simulink model "MIL_ASW"  (R2019b)
settings: Solver=FixedStepDiscrete  StartTime=0.0  StopTime=2  FixedStep=0.001  RelTol=1e-3  EnableMultiTasking=on
model workspace (MAT data in the model file):
  AccPedlCanVal : Simulink.Signal (value not decoded)
  AccPedlVal : Simulink.Signal (value not decoded)
  BrkPedlCanVal : Simulink.Signal (value not decoded)
  BrkPedlVal : Simulink.Signal (value not decoded)
  Cal1 : Simulink.Parameter (value not decoded)
  Cal10 : Simulink.Parameter (value not decoded)
  Cal11 : Simulink.Parameter (value not decoded)
  Cal12 : Simulink.Parameter (value not decoded)
  Cal2 : Simulink.Parameter (value not decoded)
  Cal3 : Simulink.Parameter (value not decoded)
  Cal4 : Simulink.Parameter (value not decoded)
  Cal5 : Simulink.Parameter (value not decoded)
  Cal6 : Simulink.Parameter (value not decoded)
  Cal7 : Simulink.Parameter (value not decoded)
  Cal8 : Simulink.Parameter (value not decoded)
  Cal9 : Simulink.Parameter (value not decoded)
  Clu1Act : Simulink.Signal (value not decoded)
  Clu1PTar : Simulink.Signal (value not decoded)
  Clu1Req : Simulink.Signal (value not decoded)
  Clu1TqTar : Simulink.Signal (value not decoded)
  Clu2Act : Simulink.Signal (value not decoded)
  Clu2PTar : Simulink.Signal (value not decoded)
  Clu2Req : Simulink.Signal (value not decoded)
  Clu2TqTar : Simulink.Signal (value not decoded)
  CluKissPtPLnch : Simulink.Parameter (value not decoded)
  CluOilTRawVal : Simulink.Signal (value not decoded)
  CluOilTVal : Simulink.Signal (value not decoded)
  CluOpenTqRatMax : Simulink.Parameter (value not decoded)
  CluPMap : Simulink.Parameter (value not decoded)
  CluPMax : Simulink.Parameter (value not decoded)
  CluPMaxGear1 : Simulink.Parameter (value not decoded)
  CluPMaxGear2 : Simulink.Parameter (value not decoded)
  CluPMaxGear3 : Simulink.Parameter (value not decoded)
  CluPMaxGear4 : Simulink.Parameter (value not decoded)
  CluPMaxGear5 : Simulink.Parameter (value not decoded)
  CluPMaxGear6 : Simulink.Parameter (value not decoded)
  CluPMaxGearR : Simulink.Parameter (value not decoded)
  CluPMin : Simulink.Parameter (value not decoded)
  CluPosnMax : Simulink.Parameter (value not decoded)
  CluSoln1IRawVal : Simulink.Signal (value not decoded)
  CluSoln1IReq : Simulink.Signal (value not decoded)
  CluSoln1IReqFlg : Simulink.Signal (value not decoded)
  CluSoln1IVal : Simulink.Signal (value not decoded)
  CluSoln1LineI : Simulink.Parameter (value not decoded)
  CluSoln1LineP : Simulink.Parameter (value not decoded)
  CluSoln1Pwm : Simulink.Signal (value not decoded)
  CluSoln2IRawVal : Simulink.Signal (value not decoded)
  CluSoln2IReq : Simulink.Signal (value not decoded)
  CluSoln2IReqFlg : Simulink.Signal (value not decoded)
  CluSoln2IVal : Simulink.Signal (value not decoded)
  CluSoln2LineI : Simulink.Parameter (value not decoded)
  CluSoln2LineP : Simulink.Parameter (value not decoded)
  CluSoln2Pwm : Simulink.Signal (value not decoded)
  CluTqMap : Simulink.Parameter (value not decoded)
  CrnkSpdRawVal : Simulink.Signal (value not decoded)
  CrnkSpdVal : Simulink.Signal (value not decoded)
  Drive_Intensity_Fuzzy : object (value not decoded)
  DrvIntenFzzy : Simulink.LookupTable (value not decoded)
  EngNIdle : Simulink.Parameter (value not decoded)
  EngNIdleMin : Simulink.Parameter (value not decoded)
  EngSpdCanVal : Simulink.Signal (value not decoded)
  EngThrCanVal : Simulink.Signal (value not decoded)
  EngTqAdd : Simulink.Parameter (value not decoded)
  EngTqCanVal : Simulink.Signal (value not decoded)
  EngTqIntvFlg : Simulink.Signal (value not decoded)
  EngTqIntvRat : Simulink.Signal (value not decoded)
  EngTqMapExtChartc : Simulink.Parameter (value not decoded)
  EngTqMapSpdIndx : Simulink.Parameter (value not decoded)
  EngTqMapThrtIndx : Simulink.Parameter (value not decoded)
  EngTqMapTqMax : Simulink.Parameter (value not decoded)
  EngTqMaxNorm : Simulink.Parameter (value not decoded)
  EngTqRef : Simulink.Parameter (value not decoded)
  EvenCluPRawVal : Simulink.Signal (value not decoded)
  EvenCluPVal : Simulink.Signal (value not decoded)
  EvenInpSpdRawVal : Simulink.Signal (value not decoded)
  EvenInpSpdVal : Simulink.Signal (value not decoded)
  FcnCallTime : Simulink.Parameter (value not decoded)
  FinalRat : Simulink.Parameter (value not decoded)
  Fork1A : Simulink.Parameter (value not decoded)
  Fork1Act : Simulink.Signal (value not decoded)
  Fork1B : Simulink.Parameter (value not decoded)
  Fork1DeltaSpdTar : Simulink.Parameter (value not decoded)
  Fork1MaxSpd1A : Simulink.Parameter (value not decoded)
  Fork1MaxSpd1B : Simulink.Parameter (value not decoded)
  Fork1MaxSpd2A : Simulink.Parameter (value not decoded)
  Fork1MaxSpd2B : Simulink.Parameter (value not decoded)
  Fork1PosnA : Simulink.Parameter (value not decoded)
  Fork1PosnB : Simulink.Parameter (value not decoded)
  Fork1PosnMaxSpd1A : Simulink.Parameter (value not decoded)
  Fork1PosnMaxSpd1B : Simulink.Parameter (value not decoded)
  Fork1PosnMaxSpd2A : Simulink.Parameter (value not decoded)
  Fork1PosnMaxSpd2B : Simulink.Parameter (value not decoded)
  Fork1PosnNeut : Simulink.Parameter (value not decoded)
  Fork1PosnNeutA : Simulink.Parameter (value not decoded)
  Fork1PosnNeutB : Simulink.Parameter (value not decoded)
  Fork1PosnRawVal : Simulink.Signal (value not decoded)
  Fork1PosnSyncA : Simulink.Parameter (value not decoded)
  Fork1PosnSyncB : Simulink.Parameter (value not decoded)
  Fork1PosnVal : Simulink.Signal (value not decoded)
  Fork1SyncTar : Simulink.Parameter (value not decoded)
  Fork2A : Simulink.Parameter (value not decoded)
  Fork2Act : Simulink.Signal (value not decoded)
  Fork2B : Simulink.Parameter (value not decoded)
  Fork2DeltaSpdTar : Simulink.Parameter (value not decoded)
  Fork2MaxSpd1A : Simulink.Parameter (value not decoded)
  Fork2MaxSpd1B : Simulink.Parameter (value not decoded)
  Fork2MaxSpd2A : Simulink.Parameter (value not decoded)
  Fork2MaxSpd2B : Simulink.Parameter (value not decoded)
  Fork2PosnA : Simulink.Parameter (value not decoded)
  Fork2PosnB : Simulink.Parameter (value not decoded)
  Fork2PosnMaxSpd1A : Simulink.Parameter (value not decoded)
  Fork2PosnMaxSpd1B : Simulink.Parameter (value not decoded)
  Fork2PosnMaxSpd2A : Simulink.Parameter (value not decoded)
  Fork2PosnMaxSpd2B : Simulink.Parameter (value not decoded)
  Fork2PosnNeut : Simulink.Parameter (value not decoded)
  Fork2PosnNeutA : Simulink.Parameter (value not decoded)
  Fork2PosnNeutB : Simulink.Parameter (value not decoded)
  Fork2PosnRawVal : Simulink.Signal (value not decoded)
  Fork2PosnSyncA : Simulink.Parameter (value not decoded)
  Fork2PosnSyncB : Simulink.Parameter (value not decoded)
  Fork2PosnVal : Simulink.Signal (value not decoded)
  Fork2SyncTar : Simulink.Parameter (value not decoded)
  Fork3A : Simulink.Parameter (value not decoded)
  Fork3Act : Simulink.Signal (value not decoded)
  Fork3B : Simulink.Parameter (value not decoded)
  Fork3DeltaSpdTar : Simulink.Parameter (value not decoded)
  Fork3MaxSpd1A : Simulink.Parameter (value not decoded)
  Fork3MaxSpd1B : Simulink.Parameter (value not decoded)
  Fork3MaxSpd2A : Simulink.Parameter (value not decoded)
  Fork3MaxSpd2B : Simulink.Parameter (value not decoded)
  Fork3PosnA : Simulink.Parameter (value not decoded)
  Fork3PosnB : Simulink.Parameter (value not decoded)
  Fork3PosnMaxSpd1A : Simulink.Parameter (value not decoded)
  Fork3PosnMaxSpd1B : Simulink.Parameter (value not decoded)
  Fork3PosnMaxSpd2A : Simulink.Parameter (value not decoded)
  Fork3PosnMaxSpd2B : Simulink.Parameter (value not decoded)
  Fork3PosnNeut : Simulink.Parameter (value not decoded)
  Fork3PosnNeutA : Simulink.Parameter (value not decoded)
  Fork3PosnNeutB : Simulink.Parameter (value not decoded)
  Fork3PosnRawVal : Simulink.Signal (value not decoded)
  Fork3PosnSyncA : Simulink.Parameter (value not decoded)
  Fork3PosnSyncB : Simulink.Parameter (value not decoded)
  Fork3PosnVal : Simulink.Signal (value not decoded)
  Fork3SyncTar : Simulink.Parameter (value not decoded)
  Fork4A : Simulink.Parameter (value not decoded)
  Fork4Act : Simulink.Signal (value not decoded)
  Fork4B : Simulink.Parameter (value not decoded)
  Fork4DeltaSpdTar : Simulink.Parameter (value not decoded)
  Fork4MaxSpd1A : Simulink.Parameter (value not decoded)
  Fork4MaxSpd1B : Simulink.Parameter (value not decoded)
  Fork4MaxSpd2A : Simulink.Parameter (value not decoded)
  Fork4MaxSpd2B : Simulink.Parameter (value not decoded)
  Fork4PosnA : Simulink.Parameter (value not decoded)
  Fork4PosnB : Simulink.Parameter (value not decoded)
  Fork4PosnMaxSpd1A : Simulink.Parameter (value not decoded)
  Fork4PosnMaxSpd1B : Simulink.Parameter (value not decoded)
  Fork4PosnMaxSpd2A : Simulink.Parameter (value not decoded)
  Fork4PosnMaxSpd2B : Simulink.Parameter (value not decoded)
  Fork4PosnNeut : Simulink.Parameter (value not decoded)
  Fork4PosnNeutA : Simulink.Parameter (value not decoded)
  Fork4PosnNeutB : Simulink.Parameter (value not decoded)
  Fork4PosnRawVal : Simulink.Signal (value not decoded)
  Fork4PosnSyncA : Simulink.Parameter (value not decoded)
  Fork4PosnSyncB : Simulink.Parameter (value not decoded)
  Fork4PosnVal : Simulink.Signal (value not decoded)
  Fork4SyncTar : Simulink.Parameter (value not decoded)
  FrntWhlRd : Simulink.Parameter (value not decoded)
  GearIdx : Simulink.Parameter (value not decoded)
  GearMax : Simulink.Parameter (value not decoded)
  GearRat : Simulink.Parameter (value not decoded)
  Launch_Engage_Fuzzy : object (value not decoded)
  LnchEngmtFzzy : Simulink.LookupTable (value not decoded)
  LubeSolnIRawVal : Simulink.Signal (value not decoded)
  LubeSolnIReq : Simulink.Signal (value not decoded)
  LubeSolnIVal : Simulink.Signal (value not decoded)
  LubeSolnLineI : Simulink.Parameter (value not decoded)
  LubeSolnLineP : Simulink.Parameter (value not decoded)
  LubeSolnPwm : Simulink.Signal (value not decoded)
  MaiLineSolnIRawVal : Simulink.Signal (value not decoded)
  MaiLineSolnIReq : Simulink.Signal (value not decoded)
  MaiLineSolnIVal : Simulink.Signal (value not decoded)
  MaiLineSolnLineI : Simulink.Parameter (value not decoded)
  MaiLineSolnLineP : Simulink.Parameter (value not decoded)
  MaiLineSolnPwm : Simulink.Signal (value not decoded)
  OddCluPRawVal : Simulink.Signal (value not decoded)
  OddCluPVal : Simulink.Signal (value not decoded)
  OddInpSpdRawVal : Simulink.Signal (value not decoded)
  OddInpSpdVal : Simulink.Signal (value not decoded)
  OutpSpdRawVal : Simulink.Signal (value not decoded)
  OutpSpdVal : Simulink.Signal (value not decoded)
  PsnsrLineP : Simulink.Parameter (value not decoded)
  PsnsrLineV : Simulink.Parameter (value not decoded)
  SftLvrCanVal : Simulink.Signal (value not decoded)
  SftLvrCfm : Simulink.Signal (value not decoded)
  SftLvrVal : Simulink.Signal (value not decoded)
  Shaft1GearAct : Simulink.Signal (value not decoded)
  Shaft1GearReq : Simulink.Signal (value not decoded)
  Shaft2GearAct : Simulink.Signal (value not decoded)
  Shaft2GearReq : Simulink.Signal (value not decoded)
  ShiftMux1SwtReq : Simulink.Signal (value not decoded)
  ShiftMux2SwtReq : Simulink.Signal (value not decoded)
  ShiftSdlEcoDwnSeln : Simulink.Parameter (value not decoded)
  ShiftSdlEcoDwnShift : Simulink.Parameter (value not decoded)
  ShiftSdlEcoUpSeln : Simulink.Parameter (value not decoded)
  ShiftSdlEcoUpShift : Simulink.Parameter (value not decoded)
  ShiftSdlPwrDwnSeln : Simulink.Parameter (value not decoded)
  ShiftSdlPwrDwnShift : Simulink.Parameter (value not decoded)
  ShiftSdlPwrUpSeln : Simulink.Parameter (value not decoded)
  ShiftSdlPwrUpShift : Simulink.Parameter (value not decoded)
  ShiftSdlSACDwnSeln : Simulink.Parameter (value not decoded)
  ShiftSdlSACDwnShift : Simulink.Parameter (value not decoded)
  ShiftSdlSACUpSeln : Simulink.Parameter (value not decoded)
  ShiftSdlSACUpShift : Simulink.Parameter (value not decoded)
  ShiftSdlThrPedlIdx : Simulink.Parameter (value not decoded)
  ShiftSoln1IRawVal : Simulink.Signal (value not decoded)
  ShiftSoln1IReq : Simulink.Signal (value not decoded)
  ShiftSoln1IVal : Simulink.Signal (value not decoded)
  ShiftSoln1LineI : Simulink.Parameter (value not decoded)
  ShiftSoln1LineP : Simulink.Parameter (value not decoded)
  ShiftSoln1Pwm : Simulink.Signal (value not decoded)
  ShiftSoln2IRawVal : Simulink.Signal (value not decoded)
  ShiftSoln2IReq : Simulink.Signal (value not decoded)
  ShiftSoln2IVal : Simulink.Signal (value not decoded)
  ShiftSoln2LineI : Simulink.Parameter (value not decoded)
  ShiftSoln2LineP : Simulink.Parameter (value not decoded)
  ShiftSoln2Pwm : Simulink.Signal (value not decoded)
  SolnOutpTRawVal : Simulink.Signal (value not decoded)
  SolnOutpTVal : Simulink.Signal (value not decoded)
  TSnsr1LineR : Simulink.Parameter (value not decoded)
  TSnsr2LineR : Simulink.Parameter (value not decoded)
  TrsmNrGearAct : Simulink.Signal (value not decoded)
  TrsmNrGearReq : Simulink.Signal (value not decoded)
  TrsmNrPreGearAct : Simulink.Signal (value not decoded)
  TrsmNrPreGearReq : Simulink.Signal (value not decoded)
  Tsnsr1LineT : Simulink.Parameter (value not decoded)
  Tsnsr2LineT : Simulink.Parameter (value not decoded)
  VehSpdCanVal : Simulink.Signal (value not decoded)
  VehSpdTrsmEstimd : Simulink.Signal (value not decoded)
  VehSpdVal : Simulink.Signal (value not decoded)
  VlvBodyTRawVal : Simulink.Signal (value not decoded)
  VlvBodyTVal : Simulink.Signal (value not decoded)
symbols that are objects in the model workspace (value not decoded): CluPMap, CluSoln1LineI, CluSoln1LineP, CluSoln2LineI, CluSoln2LineP, CluTqMap, EngNIdle, EngNIdleMin, EngTqMapThrtIndx, EngTqMapTqMax, EngTqMaxNorm, FcnCallTime, FinalRat, Fork1A, Fork1B, Fork1DeltaSpdTar, Fork1PosnA, Fork1PosnB, Fork1PosnMaxSpd1A, Fork1PosnMaxSpd1B, Fork1PosnMaxSpd2A, Fork1PosnMaxSpd2B, Fork1PosnNeut, Fork1PosnNeutA, Fork1PosnNeutB, Fork1PosnSyncA, Fork1PosnSyncB, Fork1SyncTar, Fork2A, Fork2B, Fork2DeltaSpdTar, Fork2PosnA, Fork2PosnB, Fork2PosnMaxSpd1A, Fork2PosnMaxSpd1B, Fork2PosnMaxSpd2A, Fork2PosnMaxSpd2B, Fork2PosnNeut, Fork2PosnNeutA, Fork2PosnNeutB, Fork2PosnSyncA, Fork2PosnSyncB, Fork2SyncTar, Fork3A, Fork3B, Fork3DeltaSpdTar, Fork3PosnA, Fork3PosnB, Fork3PosnMaxSpd1A, Fork3PosnMaxSpd1B, Fork3PosnMaxSpd2A, Fork3PosnMaxSpd2B, Fork3PosnNeut, Fork3PosnNeutA, Fork3PosnNeutB, Fork3PosnSyncA, Fork3PosnSyncB, Fork3SyncTar, Fork4A, Fork4B
undefined symbols (not defined in the file or in its folder): in1, out1
libraries: simulink x44, fuzblock x3
(part 9 of 10)

== stateflow chart MIL_ASW/Application_Software_SHAW/ASW_ShaftAccessControl/Chart1 ==
  state TrsmNrPreGear [parallel]
    settings: executionOrder=1
    state TrsmNrPreGearStdySt
      en:TrsmNrPreGearErrNr=0;
      TrsmNrPreGearErr=0;
    state TrsmNrPreGearProc
      state Gear0Proc [group]
        state PreGearOnShaft1And2
          en:Shaft1GearReq=TrsmNrPreGearReqLocl;
          Shaft2GearReq=TrsmNrPreGearReqLocl;
          Cntr=10;
          du:Cntr--;
        note: 
        state ErrCntShaft5
          en:ErrCntShaft++;
        state PreGearOnShaft1Req
          en:Shaft1GearReq=TrsmNrPreGearReqLocl;
          Shaft2GearReq=0;
          Cntr=10;
          du:Cntr--;
        state ErrCntShaft4
          en:ErrCntShaft++;
        state PreGearOnShaft2Req
          en:Shaft2GearReq=TrsmNrPreGearReqLocl;
          Shaft1GearReq=0;
          Cntr=10;
          du:Cntr--;
        state ErrCntShaft6
          en:ErrCntShaft++;
        PreGearOnShaft1And2 -> (junction 43) [order 1] : [Shaft1GearAct==TrsmNrPreGearReqLocl&&...
            | Shaft2GearAct==TrsmNrPreGearReqLocl]
            | {TrsmNrPreGearAct=Shaft1GearAct;
            | ErrCntShaft=0;}
        (junction 42) -> (junction 1723) [order 1] : [TrsmNrPreGearReqLocl==0]
        (junction 1723) -> PreGearOnShaft1And2 [order 1] : [Clu1Act==0&&Clu2Act==0]
            | {ErrCntShaft=0;}
        (junction 43) -> (junction 1736)
        (junction 42) -> (junction 45) [order 2]
        (junction 1723) -> (junction 1724) [order 2] : {TrsmNrPreGearErrNr=14;}
        PreGearOnShaft1And2 -> ErrCntShaft5 [order 2] : [Cntr<=0]
        ErrCntShaft5 -> PreGearOnShaft1And2 [order 1] : [ErrCntShaft<4]
        ErrCntShaft5 -> (junction 1736) [order 2] : {TrsmNrPreGearErrNr=15;
            | ErrCntShaft=0;}
        (junction 1736) -> (junction 1737)
        (junction 1724) -> (junction 1737)
        (junction 1737) -> (junction 44)
        TrsmNrPreGear.TrsmNrPreGearProc.Gear0Proc.PreGearOnShaft1Req -> (junction 44) [order 1] : [Shaft1GearAct==TrsmNrPreGearReqLocl&&...
            | Shaft2GearReq==0]
            | {TrsmNrPreGearAct=Shaft1GearAct;
            | ErrCntShaft=0;}
        (junction 45) -> (junction 46) [order 1] : [TrsmNrPreGearReqLocl==1]
        (junction 46) -> TrsmNrPreGear.TrsmNrPreGearProc.Gear0Proc.PreGearOnShaft1Req [order 1] : [Clu1Act==0&&Clu2Act==0]
            | {ErrCntShaft=0;}
        (junction 44) -> (junction 47)
        (junction 45) -> (junction 51) [order 2]
        (junction 46) -> (junction 48) [order 2] : {TrsmNrPreGearErrNr=2;}
        TrsmNrPreGear.TrsmNrPreGearProc.Gear0Proc.PreGearOnShaft1Req -> ErrCntShaft4 [order 2] : [Cntr<=0]
        ErrCntShaft4 -> TrsmNrPreGear.TrsmNrPreGearProc.Gear0Proc.PreGearOnShaft1Req [order 1] : [ErrCntShaft<4]
        ErrCntShaft4 -> (junction 47) [order 2] : {TrsmNrPreGearErrNr=3;
            | ErrCntShaft=0;}
        (junction 47) -> (junction 49)
        (junction 48) -> (junction 49)
        (junction 49) -> (junction 50)
        TrsmNrPreGear.TrsmNrPreGearProc.Gear0Proc.PreGearOnShaft2Req -> (junction 50) [order 1] : [Shaft2GearAct==TrsmNrPreGearReqLocl&&...
            | Shaft1GearReq==0]
            | {TrsmNrPreGearAct=Shaft2GearAct;
            | ErrCntShaft=0;}
        (junction 51) -> (junction 52) [order 1] : [TrsmNrPreGearReqLocl==2||...
            | TrsmNrPreGearReqLocl==7]
        (junction 52) -> TrsmNrPreGear.TrsmNrPreGearProc.Gear0Proc.PreGearOnShaft2Req [order 1] : [Clu1Act==0&&Clu2Act==0]
            | {ErrCntShaft=0;}
        (junction 50) -> (junction 53)
        (junction 51) -> (junction 56) [order 2]
        (junction 52) -> (junction 54) [order 2] : {TrsmNrPreGearErrNr=4;}
        TrsmNrPreGear.TrsmNrPreGearProc.Gear0Proc.PreGearOnShaft2Req -> ErrCntShaft6 [order 2] : [Cntr<=0]
        ErrCntShaft6 -> TrsmNrPreGear.TrsmNrPreGearProc.Gear0Proc.PreGearOnShaft2Req [order 1] : [ErrCntShaft<4]
        ErrCntShaft6 -> (junction 53) [order 2] : {TrsmNrPreGearErrNr=5;
            | ErrCntShaft=0;}
        (junction 53) -> (junction 55)
        (junction 54) -> (junction 55)
        (junction 55) -> (junction 57)
        (junction 56) -> (junction 57) : {TrsmNrPreGearErrNr=6;}
      state Ready
        en:
        TrsmNrPreGearReqLocl=TrsmNrPreGearReq;
        PreGearShiftFlg=1;
      state GearOddProc [group]
        state PreGearOnShaft2Req
          en:Shaft2GearReq=TrsmNrPreGearReqLocl;
          Cntr=10;
          du:Cntr--;
        state ErrCntShaft2
          en:ErrCntShaft++;
        (junction 95) -> (junction 96) [order 1] : [TrsmNrPreGearReqLocl==0]
            | {TrsmNrPreGearAct=TrsmNrPreGearReqLocl;}
        (junction 95) -> (junction 98) [order 2]
        (junction 96) -> (junction 97)
        (junction 98) -> (junction 97) [order 1] : [TrsmNrPreGearReqLocl==1||...
            | TrsmNrPreGearReqLocl==3||...
            | TrsmNrPreGearReqLocl==5]
            | {TrsmNrPreGearAct=TrsmNrPreGearReqLocl;}
        (junction 97) -> (junction 99)
        (junction 98) -> (junction 100) [order 2]
        TrsmNrPreGear.TrsmNrPreGearProc.GearOddProc.PreGearOnShaft2Req -> (junction 99) [order 1] : [Shaft2GearAct==TrsmNrPreGearReqLocl]
            | {TrsmNrPreGearAct=Shaft2GearAct;
            | ErrCntShaft=0;}
        (junction 100) -> (junction 101) [order 1] : [TrsmNrPreGearReqLocl==2||...
            | TrsmNrPreGearReqLocl==4||...
            | TrsmNrPreGearReqLocl==6]
        (junction 101) -> TrsmNrPreGear.TrsmNrPreGearProc.GearOddProc.PreGearOnShaft2Req [order 1] : [Clu2Act==0]
            | {ErrCntShaft=0;}
        (junction 99) -> (junction 102)
        (junction 100) -> (junction 105) [order 2]
        (junction 101) -> (junction 103) [order 2] : {TrsmNrPreGearErrNr=7;}
        TrsmNrPreGear.TrsmNrPreGearProc.GearOddProc.PreGearOnShaft2Req -> ErrCntShaft2 [order 2] : [Cntr<=0]
        ErrCntShaft2 -> TrsmNrPreGear.TrsmNrPreGearProc.GearOddProc.PreGearOnShaft2Req [order 1] : [ErrCntShaft<4]
        ErrCntShaft2 -> (junction 102) [order 2] : {TrsmNrPreGearErrNr=8;
            | ErrCntShaft=0;}
        (junction 102) -> (junction 104)
        (junction 103) -> (junction 104)
        (junction 104) -> (junction 106)
        (junction 105) -> (junction 106) : {TrsmNrPreGearErrNr=9;}
      state GearEvenProc [group]
        state PreGearOnShaft1Req
          en:Shaft1GearReq=TrsmNrPreGearReqLocl;
          Cntr=10;
          du:Cntr--;
        state ErrCntShaft1
          en:ErrCntShaft++;
        (junction 132) -> (junction 133) [order 1] : [TrsmNrPreGearReqLocl==0]
            | {TrsmNrPreGearAct=TrsmNrPreGearReqLocl;}
        (junction 132) -> (junction 135) [order 2]
        (junction 133) -> (junction 134)
        TrsmNrPreGear.TrsmNrPreGearProc.GearEvenProc.PreGearOnShaft1Req -> (junction 134) [order 1] : [Shaft1GearAct==TrsmNrPreGearReqLocl]
            | {TrsmNrPreGearAct=Shaft1GearAct;
            | ErrCntShaft=0;}
        (junction 135) -> (junction 136) [order 1] : [TrsmNrPreGearReqLocl==1||...
            | TrsmNrPreGearReqLocl==3||...
            | TrsmNrPreGearReqLocl==5]
        (junction 136) -> TrsmNrPreGear.TrsmNrPreGearProc.GearEvenProc.PreGearOnShaft1Req [order 1] : [Clu1Act==0]
            | {ErrCntShaft=0;}
        (junction 134) -> (junction 137)
        (junction 135) -> (junction 141) [order 2]
        (junction 136) -> (junction 138) [order 2] : {TrsmNrPreGearErrNr=10;}
        TrsmNrPreGear.TrsmNrPreGearProc.GearEvenProc.PreGearOnShaft1Req -> ErrCntShaft1 [order 2] : [Cntr<=0]
        ErrCntShaft1 -> TrsmNrPreGear.TrsmNrPreGearProc.GearEvenProc.PreGearOnShaft1Req [order 1] : [ErrCntShaft<4]
        ErrCntShaft1 -> (junction 137) [order 2] : {TrsmNrPreGearErrNr=11;
            | ErrCntShaft=0;}
        (junction 137) -> (junction 139)
        (junction 138) -> (junction 139)
        (junction 139) -> (junction 140)
        (junction 141) -> (junction 140) [order 1] : [TrsmNrPreGearReqLocl==2||...
            | TrsmNrPreGearReqLocl==4||...
            | TrsmNrPreGearReqLocl==6]
            | {TrsmNrPreGearAct=TrsmNrPreGearReqLocl;}
        (junction 141) -> (junction 142) [order 2]
        (junction 140) -> (junction 143)
        (junction 142) -> (junction 143) : {TrsmNrPreGearErrNr=12;}
      state GearRvsProc [group]
        (junction 169) -> (junction 170) [order 1] : [TrsmNrPreGearReqLocl==0]
            | {TrsmNrPreGearAct=TrsmNrPreGearReqLocl;}
        (junction 169) -> (junction 172) [order 2]
        (junction 170) -> (junction 171)
        (junction 172) -> (junction 171) [order 1] : [TrsmNrPreGearReqLocl==7]
        (junction 171) -> (junction 1662)
        (junction 172) -> (junction 1660) [order 2]
        (junction 1660) -> (junction 1662) : {TrsmNrPreGearErrNr=13;}
      state end
      TrsmNrPreGear.TrsmNrPreGearProc.Ready -> (junction 42) [order 1] : [TrsmNrGearAct==0]
      TrsmNrPreGear.TrsmNrPreGearProc.Ready -> (junction 132) [order 3] : [TrsmNrGearAct==2||...
          | TrsmNrGearAct==4||...
          | TrsmNrGearAct==6]
      (junction 57) -> (junction 4)
      TrsmNrPreGear.TrsmNrPreGearProc.Ready -> (junction 95) [order 2] : [TrsmNrGearAct==1||...
          | TrsmNrGearAct==3||...
          | TrsmNrGearAct==5]
      (junction 106) -> (junction 6)
      (junction 4) -> (junction 6)
      (junction 143) -> (junction 8)
      (default) -> TrsmNrPreGear.TrsmNrPreGearProc.Ready
      (junction 6) -> (junction 8)
      (junction 8) -> (junction 10)
      (junction 10) -> (junction 1607)
      (junction 1662) -> (junction 10)
      TrsmNrPreGear.TrsmNrPreGearProc.Ready -> (junction 169) [order 4] : [TrsmNrGearAct==7]
      TrsmNrPreGear.TrsmNrPreGearProc.Ready -> TrsmNrPreGear.TrsmNrPreGearProc.end [order 5] : {TrsmNrPreGearErrNr=1;}
      (junction 1607) -> TrsmNrPreGear.TrsmNrPreGearProc.end
      TrsmNrPreGear.TrsmNrPreGearProc.end -> TrsmNrPreGearProc : [TrsmNrPreGearErrNr>0]
          | {TrsmNrPreGearErr++;
          | TrsmNrPreGearErrNr=0;}
    (default) -> TrsmNrPreGearStdySt
    TrsmNrPreGearStdySt -> (junction 1945) [order 1] : [TrsmNrPreGearAct!=TrsmNrPreGearReq]
    (junction 1945) -> TrsmNrPreGearProc : [GearShiftFlg==0]
    (junction 1947) -> (junction 1945)
    TrsmNrPreGearStdySt -> (junction 1947) [order 2] : [Shaft1GearAct!=TrsmNrPreGearReq&&...
        | Shaft2GearAct!=TrsmNrPreGearReq]
    (junction 1952) -> (junction 1947)
    TrsmNrPreGearStdySt -> (junction 1952) [order 3] : [TrsmNrPreGearReq==0&&...
        | (Shaft1GearAct!=0||Shaft2GearAct!=0)]
    TrsmNrPreGearProc -> TrsmNrPreGearStdySt : [TrsmNrPreGearAct==TrsmNrPreGearReqLocl]
        | {PreGearShiftFlg=0;}
  state TrsmNrGear [parallel]
    settings: executionOrder=2
    state TrsmNrGearStdySt
      en:TrsmNrGearErrNr=0;
      TrsmNrGearErr=0;
    state TrsmNrGearProc
      state Ready
        en:
        TrsmNrGearReqLocl=TrsmNrGearReq;
        GearShiftFlg=1;
      state Gear0Proc [group]
        state ErrCluCnt8
          en:ErrCntGear++;
        state Clu1DisengdClu2Disengd
          en:Clu1Req=0;
          Clu2Req=0;
          Cntr=10;
          du:Cntr--;
        state ErrCluCnt1
          en:ErrCntGear++;
        state ErrCluCnt2
          en:ErrCntGear++;
        state ErrCluCnt3
          en:ErrCntGear++;
        state Clu1EngdClu2Disengd
          en:Clu1Req=1;
          Clu2Req=0;
          Cntr=10;
          du:Cntr--;
        state ChkPreGearOnShaft1
          en:Shaft1GearReq=TrsmNrGearReqLocl;
          Cntr=10;
          du:Cntr--;
        state Set0OnShaft2
          en:Shaft2GearReq=0;
          Cntr=10;
          du:Cntr--;
        state ErrCluCnt11
          en:ErrCntGear++;
        state ErrCluCnt9
          en:ErrCntGear++;
        state ErrCluCnt10
          en:ErrCntGear++;
        state Set0OnShaftR
          en:Shaft1GearReq=0;
          Cntr=10;
          du:Cntr--;
        state Clu1EngdClu2Disengd1
          en:Clu1Req=1;
          Clu2Req=0;
          Cntr=10;
          du:Cntr--;
        state ChkPreGearOnShaftR
          en:Shaft2GearReq=TrsmNrGearReqLocl;
          Cntr=10;
          du:Cntr--;
        state ErrCluCnt5
          en:ErrCntGear++;
        state ErrCluCnt6
          en:ErrCntGear++;
        state ErrCluCnt4
          en:ErrCntGear++;
        state ChkPreGearOnShaft2
          en:Shaft2GearReq=TrsmNrGearReqLocl;
          Cntr=10;
          du:Cntr--;
        state Clu1DisengdClu2Engd
          en:Clu1Req=0;
          Clu2Req=1;
          Cntr=10;
          du:Cntr--;
        state Set0OnShaft1
          en:Shaft1GearReq=0;
          Cntr=10;
          du:Cntr--;
        (junction 1747) -> (junction 1748)
        (junction 1748) -> (junction 1762)
        TrsmNrGear.TrsmNrGearProc.Gear0Proc.ErrCluCnt8 -> (junction 1747) [order 2] : {TrsmNrGearErrNr=30;
            | ErrCntGear=0;}
        (junction 1762) -> (junction 1761)
        TrsmNrGear.TrsmNrGearProc.Gear0Proc.Clu1DisengdClu2Disengd -> TrsmNrGear.TrsmNrGearProc.Gear0Proc.ErrCluCnt8 [order 2] : [Cntr<=0]
        TrsmNrGear.TrsmNrGearProc.Gear0Proc.ErrCluCnt8 -> TrsmNrGear.TrsmNrGearProc.Gear0Proc.Clu1DisengdClu2Disengd [order 1] : [ErrCntGear<40]
        (junction 221) -> TrsmNrGear.TrsmNrGearProc.Gear0Proc.Clu1DisengdClu2Disengd [order 1] : [TrsmNrGearReq==0]
            | {ErrCntGear=0;}
        TrsmNrGear.TrsmNrGearProc.Gear0Proc.Clu1DisengdClu2Disengd -> (junction 1939) [order 1] : [Clu1Act==0&&Clu2Act==0]
            | {ErrCntGear=0;}
        (junction 1939) -> (junction 1761) : {TrsmNrGearAct=TrsmNrGearReqLocl;
            | ErrCntGear=0;}
        (junction 221) -> (junction 227) [order 2]
        (junction 1761) -> (junction 225)
        (junction 223) -> (junction 224)
        (junction 224) -> (junction 225)
        (junction 222) -> (junction 223)
        ErrCluCnt2 -> (junction 223) [order 2] : {TrsmNrGearErrNr=3;
            | ErrCntGear=0;}
        ErrCluCnt3 -> (junction 224) [order 2] : {TrsmNrGearErrNr=4;
            | ErrCntGear=0;}
        (junction 225) -> (junction 226)
        ErrCluCnt1 -> (junction 222) [order 2] : {TrsmNrGearErrNr=2;
            | ErrCntGear=0;}
        TrsmNrGear.TrsmNrGearProc.Gear0Proc.ChkPreGearOnShaft1 -> ErrCluCnt1 [order 2] : [Cntr<=0]
        ErrCluCnt1 -> TrsmNrGear.TrsmNrGearProc.Gear0Proc.ChkPreGearOnShaft1 [order 1] : [ErrCntGear<4]
        TrsmNrGear.TrsmNrGearProc.Gear0Proc.Clu1EngdClu2Disengd -> ErrCluCnt2 [order 2] : [Cntr<=0]
        ErrCluCnt2 -> TrsmNrGear.TrsmNrGearProc.Gear0Proc.Clu1EngdClu2Disengd [order 1] : [ErrCntGear<40]
        TrsmNrGear.TrsmNrGearProc.Gear0Proc.Set0OnShaft2 -> ErrCluCnt3 [order 2] : [Cntr<=0]
        ErrCluCnt3 -> TrsmNrGear.TrsmNrGearProc.Gear0Proc.Set0OnShaft2 [order 1] : [ErrCntGear<4]
        TrsmNrGear.TrsmNrGearProc.Gear0Proc.Set0OnShaft2 -> (junction 226) [order 1] : [Shaft2GearAct==0]
            | {TrsmNrGearAct=TrsmNrGearReqLocl;
            | TrsmNrPreGearAct=TrsmNrGearAct;
            | ErrCntGear=0;}
        (junction 227) -> TrsmNrGear.TrsmNrGearProc.Gear0Proc.ChkPreGearOnShaft1 [order 1] : [TrsmNrGearReqLocl==1||...
            | TrsmNrGearReqLocl==3||...
            | TrsmNrGearReqLocl==5]
            | {ErrCntGear=0;}
        TrsmNrGear.TrsmNrGearProc.Gear0Proc.Clu1EngdClu2Disengd -> TrsmNrGear.TrsmNrGearProc.Gear0Proc.Set0OnShaft2 [order 1] : [Clu1Act==1&&Clu2Act==0]
            | {ErrCntGear=0;}
        TrsmNrGear.TrsmNrGearProc.Gear0Proc.ChkPreGearOnShaft1 -> TrsmNrGear.TrsmNrGearProc.Gear0Proc.Clu1EngdClu2Disengd [order 1] : [TrsmNrPreGearAct==TrsmNrGearReqLocl||...
            | Shaft1GearAct==TrsmNrGearReqLocl]
            | {TrsmNrPreGearAct=TrsmNrGearReqLocl;
            | ErrCntGear=0;}
        (junction 226) -> (junction 1931)
        (junction 227) -> (junction 1904) [order 2]
        (junction 1922) -> (junction 1928)
        (junction 1928) -> (junction 1931)
        (junction 1921) -> (junction 1922)
        TrsmNrGear.TrsmNrGearProc.Gear0Proc.ErrCluCnt10 -> (junction 1922) [order 2] : {TrsmNrGearErrNr=3;
            | ErrCntGear=0;}
        TrsmNrGear.TrsmNrGearProc.Gear0Proc.ErrCluCnt11 -> (junction 1928) [order 2] : {TrsmNrGearErrNr=7;
            | ErrCntGear=0;}
        (junction 1931) -> (junction 1932)
        TrsmNrGear.TrsmNrGearProc.Gear0Proc.ErrCluCnt9 -> (junction 1921) [order 2] : {TrsmNrGearErrNr=2;
            | ErrCntGear=0;}
        Set0OnShaftR -> TrsmNrGear.TrsmNrGearProc.Gear0Proc.ErrCluCnt11 [order 1] : [Cntr<=0]
        TrsmNrGear.TrsmNrGearProc.Gear0Proc.ErrCluCnt11 -> Set0OnShaftR [order 1] : [ErrCntGear<4]
        TrsmNrGear.TrsmNrGearProc.Gear0Proc.ErrCluCnt9 -> ChkPreGearOnShaftR [order 1] : [ErrCntGear<4]
        ChkPreGearOnShaftR -> TrsmNrGear.TrsmNrGearProc.Gear0Proc.ErrCluCnt9 [order 2] : [Cntr<=0]
        Clu1EngdClu2Disengd1 -> TrsmNrGear.TrsmNrGearProc.Gear0Proc.ErrCluCnt10 [order 2] : [Cntr<=0]
        TrsmNrGear.TrsmNrGearProc.Gear0Proc.ErrCluCnt10 -> Clu1EngdClu2Disengd1 [order 1] : [ErrCntGear<40]
        Set0OnShaftR -> (junction 1932) [order 2] : [Shaft1GearAct==0]
            | {TrsmNrGearAct=TrsmNrGearReqLocl;
            | TrsmNrPreGearAct=TrsmNrGearAct;
            | ErrCntGear=0;}
        (junction 1904) -> ChkPreGearOnShaftR [order 1] : [TrsmNrGearReqLocl==7]
            | {ErrCntGear=0;}
        Clu1EngdClu2Disengd1 -> Set0OnShaftR [order 1] : [Clu1Act==1&&Clu2Act==0]
            | {ErrCntGear=0;}
        ChkPreGearOnShaftR -> Clu1EngdClu2Disengd1 [order 1] : [TrsmNrPreGearAct==TrsmNrGearReqLocl||...
            | Shaft2GearAct==TrsmNrGearReqLocl]
            | {TrsmNrPreGearAct=TrsmNrGearReqLocl;
            | ErrCntGear=0;}
        (junction 1932) -> (junction 228)
        (junction 1904) -> (junction 232) [order 2]
        (junction 230) -> (junction 231)
        (junction 231) -> (junction 228)
        (junction 229) -> (junction 230)
        ErrCluCnt6 -> (junction 231) [order 2] : {TrsmNrGearErrNr=7;
            | ErrCntGear=0;}
        (junction 228) -> (junction 233)
        TrsmNrGear.TrsmNrGearProc.Gear0Proc.ErrCluCnt5 -> (junction 229) [order 2] : {TrsmNrGearErrNr=5;
            | ErrCntGear=0;}
        TrsmNrGear.TrsmNrGearProc.Gear0Proc.ErrCluCnt4 -> (junction 230) [order 2] : {TrsmNrGearErrNr=6;
            | ErrCntGear=0;}
        TrsmNrGear.TrsmNrGearProc.Gear0Proc.ChkPreGearOnShaft2 -> TrsmNrGear.TrsmNrGearProc.Gear0Proc.ErrCluCnt5 [order 2] : [Cntr<=0]
        TrsmNrGear.TrsmNrGearProc.Gear0Proc.ErrCluCnt5 -> TrsmNrGear.TrsmNrGearProc.Gear0Proc.ChkPreGearOnShaft2 [order 1] : [ErrCntGear<4]
        TrsmNrGear.TrsmNrGearProc.Gear0Proc.Set0OnShaft1 -> ErrCluCnt6 [order 2] : [Cntr<=0]
        ErrCluCnt6 -> TrsmNrGear.TrsmNrGearProc.Gear0Proc.Set0OnShaft1 [order 1] : [ErrCntGear<4]
        TrsmNrGear.TrsmNrGearProc.Gear0Proc.Clu1DisengdClu2Engd -> TrsmNrGear.TrsmNrGearProc.Gear0Proc.ErrCluCnt4 [order 2] : [Cntr<=0]
        TrsmNrGear.TrsmNrGearProc.Gear0Proc.ErrCluCnt4 -> TrsmNrGear.TrsmNrGearProc.Gear0Proc.Clu1DisengdClu2Engd [order 1] : [ErrCntGear<40]
        (junction 232) -> TrsmNrGear.TrsmNrGearProc.Gear0Proc.ChkPreGearOnShaft2 [order 1] : [TrsmNrGearReqLocl==2||...
            | TrsmNrGearReqLocl==4||...
            | TrsmNrGearReqLocl==6]
            | {ErrCntGear=0;}
        TrsmNrGear.TrsmNrGearProc.Gear0Proc.ChkPreGearOnShaft2 -> TrsmNrGear.TrsmNrGearProc.Gear0Proc.Clu1DisengdClu2Engd [order 1] : [TrsmNrPreGearAct==TrsmNrGearReqLocl||...
            | Shaft2GearAct==TrsmNrGearReqLocl]
            | {TrsmNrPreGearAct=TrsmNrGearReqLocl;
            | ErrCntGear=0;}
        (junction 232) -> (junction 234) [order 2]
        TrsmNrGear.TrsmNrGearProc.Gear0Proc.Set0OnShaft1 -> (junction 233) [order 1] : [Shaft1GearAct==0]
            | {TrsmNrGearAct=TrsmNrGearReqLocl;
            | TrsmNrPreGearAct=TrsmNrGearAct;
            | ErrCntGear=0;}
        TrsmNrGear.TrsmNrGearProc.Gear0Proc.Clu1DisengdClu2Engd -> TrsmNrGear.TrsmNrGearProc.Gear0Proc.Set0OnShaft1 [order 1] : [Clu1Act==0&&Clu2Act==1]
            | {ErrCntGear=0;}
        (junction 233) -> (junction 235)
        (junction 234) -> (junction 235) : {TrsmNrGearErrNr=8;}
      state GearOddProc [group]
        state ErrCluCnt4
          en:ErrCntGear++;
        state Clu1DisengdClu2Disengd
          en:Clu1Req=0;
          Clu2Req=0;
          Cntr=10;
          du:Cntr--;
        state ErrCluCnt7
          en:ErrCntGear++;
        state ErrCluCnt8
          en:ErrCntGear++;
        state ErrCluCnt9
          en:ErrCntGear++;
        state Clu1Disengd
          en:Clu1Req=0;
          Clu2Req=0;
          Cntr=10;
          du:Cntr--;
        state ChgOnShaft1
          en:Shaft1GearReq=TrsmNrGearReqLocl;
          Shaft2GearReq=0;
          Cntr=10;
          du:Cntr--;
        state Clu1Engd
          en:Clu1Req=1;
          Clu2Req=0;
          Cntr=10;
          du:Cntr--;
        state ErrCluCnt5
          en:ErrCntGear++;
        state ErrCluCnt10
          en:ErrCntGear++;
        state ErrCluCnt11
          en:ErrCntGear++;
        state Clu1DisengdClu2Engd
          en:Clu1Req=0;
          Clu2Req=1;
          Cntr=10;
          du:Cntr--;
        state ChkPreGearOnShaft2
          en:Shaft2GearReq=TrsmNrGearReqLocl;
          Cntr=10;
          du:Cntr--;
        state Set0OnShaft1
          en:Shaft1GearReq=0;
          Cntr=10;
          du:Cntr--;
        (junction 295) -> (junction 296)
        (junction 294) -> (junction 295)
        TrsmNrGear.TrsmNrGearProc.GearOddProc.ErrCluCnt4 -> (junction 294) [order 2] : {TrsmNrGearErrNr=9;
            | ErrCntGear=0;}
        (junction 296) -> (junction 298)
        TrsmNrGear.TrsmNrGearProc.GearOddProc.Clu1DisengdClu2Disengd -> TrsmNrGear.TrsmNrGearProc.GearOddProc.ErrCluCnt4 [order 2] : [Cntr<=0]
        TrsmNrGear.TrsmNrGearProc.GearOddProc.ErrCluCnt4 -> TrsmNrGear.TrsmNrGearProc.GearOddProc.Clu1DisengdClu2Disengd [order 1] : [ErrCntGear<40]
        (junction 297) -> TrsmNrGear.TrsmNrGearProc.GearOddProc.Clu1DisengdClu2Disengd [order 1] : [TrsmNrGearReqLocl==0]
            | {ErrCntGear=0;}
        TrsmNrGear.TrsmNrGearProc.GearOddProc.Clu1DisengdClu2Disengd -> (junction 1940) [order 1] : [Clu1Act==0&&Clu2Act==0]
            | {ErrCntGear=0;}
        (junction 1940) -> (junction 298) : {TrsmNrGearAct=TrsmNrGearReqLocl;
            | ErrCntGear=0;}
        (junction 297) -> (junction 303) [order 2]
        (junction 298) -> (junction 301)
        (junction 299) -> (junction 302)
        (junction 302) -> (junction 300)
        (junction 300) -> (junction 301)
        TrsmNrGear.TrsmNrGearProc.GearOddProc.ErrCluCnt7 -> (junction 299) [order 2] : {TrsmNrGearErrNr=11;
            | ErrCntGear=0;}
        TrsmNrGear.TrsmNrGearProc.GearOddProc.ErrCluCnt8 -> (junction 302) [order 2] : {TrsmNrGearErrNr=12;
            | ErrCntGear=0;}
        TrsmNrGear.TrsmNrGearProc.GearOddProc.ErrCluCnt9 -> (junction 300) [order 2] : {TrsmNrGearErrNr=13;
            | ErrCntGear=0;}
        (junction 301) -> (junction 304)
        Clu1Disengd -> TrsmNrGear.TrsmNrGearProc.GearOddProc.ErrCluCnt7 [order 2] : [Cntr<=0]
        TrsmNrGear.TrsmNrGearProc.GearOddProc.ErrCluCnt7 -> Clu1Disengd [order 1] : [ErrCntGear<40]
        ChgOnShaft1 -> TrsmNrGear.TrsmNrGearProc.GearOddProc.ErrCluCnt8 [order 2] : [Cntr<=0]
        TrsmNrGear.TrsmNrGearProc.GearOddProc.ErrCluCnt8 -> ChgOnShaft1 [order 1] : [ErrCntGear<4]
        TrsmNrGear.TrsmNrGearProc.GearOddProc.Clu1Engd -> TrsmNrGear.TrsmNrGearProc.GearOddProc.ErrCluCnt9 [order 2] : [Cntr<=0]
        TrsmNrGear.TrsmNrGearProc.GearOddProc.ErrCluCnt9 -> TrsmNrGear.TrsmNrGearProc.GearOddProc.Clu1Engd [order 1] : [ErrCntGear<40]
        (junction 303) -> (junction 1631) [order 1] : [TrsmNrGearReqLocl==1||...
            | TrsmNrGearReqLocl==3||...
            | TrsmNrGearReqLocl==5]
            | {ErrCntGear=0;}
        (junction 1631) -> Clu1Disengd
        ChgOnShaft1 -> TrsmNrGear.TrsmNrGearProc.GearOddProc.Clu1Engd [order 1] : [Shaft1GearAct==TrsmNrGearReqLocl&&...
            | Shaft2GearAct==0]
            | {TrsmNrPreGearAct=TrsmNrGearReqLocl;
            | ErrCntGear=0;}
        (junction 303) -> (junction 310) [order 2]
        Clu1Disengd -> ChgOnShaft1 [order 1] : [Clu1Act==0&&...
            | Clu2Act==0]
            | {ErrCntGear=0;}
        TrsmNrGear.TrsmNrGearProc.GearOddProc.Clu1Engd -> (junction 304) [order 1] : [Clu1Act==1&&...
            | Clu2Act==0]
            | {TrsmNrGearAct=TrsmNrGearReqLocl;
            | ErrCntGear=0;}
        (junction 304) -> (junction 1636)
        (junction 1636) -> (junction 306)
        (junction 308) -> (junction 305)
        (junction 305) -> (junction 306)
        (junction 307) -> (junction 308)
        TrsmNrGear.TrsmNrGearProc.GearOddProc.ErrCluCnt10 -> (junction 308) [order 2] : {TrsmNrGearErrNr=15;
            | ErrCntGear=0;}
        TrsmNrGear.TrsmNrGearProc.GearOddProc.ErrCluCnt11 -> (junction 305) [order 2] : {TrsmNrGearErrNr=16;
            | ErrCntGear=0;}
        (junction 306) -> (junction 309)
        TrsmNrGear.TrsmNrGearProc.GearOddProc.ErrCluCnt5 -> (junction 307) [order 2] : {TrsmNrGearErrNr=14;
            | ErrCntGear=0;}
        TrsmNrGear.TrsmNrGearProc.GearOddProc.ChkPreGearOnShaft2 -> TrsmNrGear.TrsmNrGearProc.GearOddProc.ErrCluCnt5 [order 2] : [Cntr<=0]
        TrsmNrGear.TrsmNrGearProc.GearOddProc.ErrCluCnt5 -> TrsmNrGear.TrsmNrGearProc.GearOddProc.ChkPreGearOnShaft2 [order 1] : [ErrCntGear<4]
        TrsmNrGear.TrsmNrGearProc.GearOddProc.Clu1DisengdClu2Engd -> TrsmNrGear.TrsmNrGearProc.GearOddProc.ErrCluCnt10 [order 2] : [Cntr<=0]
        TrsmNrGear.TrsmNrGearProc.GearOddProc.ErrCluCnt10 -> TrsmNrGear.TrsmNrGearProc.GearOddProc.Clu1DisengdClu2Engd [order 1] : [ErrCntGear<40]
        TrsmNrGear.TrsmNrGearProc.GearOddProc.Set0OnShaft1 -> TrsmNrGear.TrsmNrGearProc.GearOddProc.ErrCluCnt11 [order 2] : [Cntr<=0]
        TrsmNrGear.TrsmNrGearProc.GearOddProc.ErrCluCnt11 -> TrsmNrGear.TrsmNrGearProc.GearOddProc.Set0OnShaft1 [order 1] : [ErrCntGear<4]
        TrsmNrGear.TrsmNrGearProc.GearOddProc.ChkPreGearOnShaft2 -> TrsmNrGear.TrsmNrGearProc.GearOddProc.Clu1DisengdClu2Engd [order 1] : [TrsmNrPreGearAct==TrsmNrGearReqLocl||...
            | Shaft2GearAct==TrsmNrGearReqLocl]
            | {TrsmNrPreGearAct=TrsmNrGearReqLocl;
            | ErrCntGear=0;}
        TrsmNrGear.TrsmNrGearProc.GearOddProc.Set0OnShaft1 -> (junction 309) [order 1] : [Shaft1GearAct==0]
            | {TrsmNrGearAct=TrsmNrGearReqLocl;
            | TrsmNrPreGearAct=TrsmNrGearAct;
            | ErrCntGear=0;}
        (junction 310) -> TrsmNrGear.TrsmNrGearProc.GearOddProc.ChkPreGearOnShaft2 [order 1] : [TrsmNrGearReqLocl==2||...
            | TrsmNrGearReqLocl==4||...
            | TrsmNrGearReqLocl==6]
            | {ErrCntGear=0;}
        TrsmNrGear.TrsmNrGearProc.GearOddProc.Clu1DisengdClu2Engd -> TrsmNrGear.TrsmNrGearProc.GearOddProc.Set0OnShaft1 [order 1] : [Clu1Act==0&&Clu2Act==1]
            | {ErrCntGear=0;}
        (junction 309) -> (junction 312)
        (junction 310) -> (junction 311) [order 2]
        (junction 311) -> (junction 312) : {TrsmNrGearErrNr=17;}
      state GearEvenProc [group]
        state ErrCluCnt4
          en:ErrCntGear++;
        state Clu1DisengdClu2Disengd
          en:Clu1Req=0;
          Clu2Req=0;
          Cntr=10;
          du:Cntr--;
        state ErrCluCnt9
          en:ErrCntGear++;
        state ErrCluCnt7
          en:ErrCntGear++;
        state ErrCluCnt8
          en:ErrCntGear++;
        state Clu2Disengd
          en:Clu1Req=0;
          Clu2Req=0;
          Cntr=10;
          du:Cntr--;
        state Clu1Engd
          en:Clu1Req=0;
          Clu2Req=1;
          Cntr=10;
          du:Cntr--;
        state ChgOnShaft2
          en:Shaft1GearReq=0;
          Shaft2GearReq=TrsmNrGearReqLocl;
          Cntr=10;
          du:Cntr--;
        state ErrCluCnt5
          en:ErrCntGear++;
        state ErrCluCnt11
          en:ErrCntGear++;
        state ErrCluCnt10
          en:ErrCntGear++;
        state ChkPreGearOnShaft1
          en:Shaft1GearReq=TrsmNrGearReqLocl;
          Cntr=10;
          du:Cntr--;
        state Clu1EngdClu2Disengd
          en:Clu1Req=1;
          Clu2Req=0;
          Cntr=10;
          du:Cntr--;
        state Set0OnShaft2
          en:Shaft2GearReq=0;
          Cntr=10;
          du:Cntr--;
        (junction 386) -> (junction 387)
        (junction 387) -> (junction 388) : {ErrCntGear=0;}
        TrsmNrGear.TrsmNrGearProc.GearEvenProc.ErrCluCnt4 -> (junction 386) [order 2] : {TrsmNrGearErrNr=18;}
        (junction 388) -> (junction 390)
        TrsmNrGear.TrsmNrGearProc.GearEvenProc.Clu1DisengdClu2Disengd -> TrsmNrGear.TrsmNrGearProc.GearEvenProc.ErrCluCnt4 [order 2] : [Cntr<=0]
        TrsmNrGear.TrsmNrGearProc.GearEvenProc.ErrCluCnt4 -> TrsmNrGear.TrsmNrGearProc.GearEvenProc.Clu1DisengdClu2Disengd [order 1] : [ErrCntGear<40]
        TrsmNrGear.TrsmNrGearProc.GearEvenProc.Clu1DisengdClu2Disengd -> (junction 1941) [order 1] : [Clu1Act==0&&Clu2Act==0]
            | {ErrCntGear=0;}
        (junction 1941) -> (junction 390) : {TrsmNrGearAct=TrsmNrGearReqLocl;
            | ErrCntGear=0;}
        (junction 389) -> TrsmNrGear.TrsmNrGearProc.GearEvenProc.Clu1DisengdClu2Disengd [order 1] : [TrsmNrGearReqLocl==0]
            | {ErrCntGear=0;}
        (junction 390) -> (junction 394)
        (junction 389) -> (junction 395) [order 2]
        (junction 391) -> (junction 392)
        (junction 392) -> (junction 393)
        (junction 393) -> (junction 394) : {ErrCntGear=0;}
        TrsmNrGear.TrsmNrGearProc.GearEvenProc.ErrCluCnt7 -> (junction 391) [order 2] : {TrsmNrGearErrNr=20;}
        TrsmNrGear.TrsmNrGearProc.GearEvenProc.ErrCluCnt8 -> (junction 392) [order 2] : {TrsmNrGearErrNr=21;}
        TrsmNrGear.TrsmNrGearProc.GearEvenProc.ErrCluCnt9 -> (junction 393) [order 2] : {TrsmNrGearErrNr=22;}
        (junction 394) -> (junction 396)
        TrsmNrGear.TrsmNrGearProc.GearEvenProc.Clu1Engd -> TrsmNrGear.TrsmNrGearProc.GearEvenProc.ErrCluCnt9 [order 2] : [Cntr<=0]
        TrsmNrGear.TrsmNrGearProc.GearEvenProc.ErrCluCnt9 -> TrsmNrGear.TrsmNrGearProc.GearEvenProc.Clu1Engd [order 1] : [ErrCntGear<40]
        Clu2Disengd -> TrsmNrGear.TrsmNrGearProc.GearEvenProc.ErrCluCnt7 [order 2] : [Cntr<=0]
        TrsmNrGear.TrsmNrGearProc.GearEvenProc.ErrCluCnt7 -> Clu2Disengd [order 1] : [ErrCntGear<40]
        ChgOnShaft2 -> TrsmNrGear.TrsmNrGearProc.GearEvenProc.ErrCluCnt8 [order 2] : [Cntr<=0]
        TrsmNrGear.TrsmNrGearProc.GearEvenProc.ErrCluCnt8 -> ChgOnShaft2 [order 1] : [ErrCntGear<4]
        (junction 395) -> (junction 1642) [order 1] : [TrsmNrGearReqLocl==2||...
            | TrsmNrGearReqLocl==4||...
            | TrsmNrGearReqLocl==6]
            | {ErrCntGear=0;}
        (junction 1642) -> Clu2Disengd
        Clu2Disengd -> ChgOnShaft2 [order 1] : [Clu1Act==0&&...
            | Clu2Act==0]
            | {ErrCntGear=0;}
        (junction 395) -> (junction 402) [order 2]
        TrsmNrGear.TrsmNrGearProc.GearEvenProc.Clu1Engd -> (junction 396) [order 1] : [Clu1Act==0&&...
            | Clu2Act==1]
            | {TrsmNrGearAct=TrsmNrGearReqLocl;
            | TrsmNrPreGearAct=TrsmNrGearAct;
            | ErrCntGear=0;}
        ChgOnShaft2 -> TrsmNrGear.TrsmNrGearProc.GearEvenProc.Clu1Engd [order 1] : [Shaft2GearAct==TrsmNrGearReqLocl&&...
            | Shaft1GearAct==0]
            | {TrsmNrPreGearAct=TrsmNrGearReqLocl;
            | ErrCntGear=0;}
        (junction 396) -> (junction 1646)
        (junction 1646) -> (junction 398)
        (junction 400) -> (junction 397)
        (junction 399) -> (junction 400)
        (junction 397) -> (junction 398) : {ErrCntGear=0;}
        TrsmNrGear.TrsmNrGearProc.GearEvenProc.ErrCluCnt10 -> (junction 400) [order 2] : {TrsmNrGearErrNr=24;}
        TrsmNrGear.TrsmNrGearProc.GearEvenProc.ErrCluCnt11 -> (junction 397) [order 2] : {TrsmNrGearErrNr=25;}
        (junction 398) -> (junction 401)
        TrsmNrGear.TrsmNrGearProc.GearEvenProc.ErrCluCnt5 -> (junction 399) [order 2] : {TrsmNrGearErrNr=23;}
        TrsmNrGear.TrsmNrGearProc.GearEvenProc.ChkPreGearOnShaft1 -> TrsmNrGear.TrsmNrGearProc.GearEvenProc.ErrCluCnt5 [order 2] : [Cntr<=0]
        TrsmNrGear.TrsmNrGearProc.GearEvenProc.ErrCluCnt5 -> TrsmNrGear.TrsmNrGearProc.GearEvenProc.ChkPreGearOnShaft1 [order 1] : [ErrCntGear<4]
        TrsmNrGear.TrsmNrGearProc.GearEvenProc.Set0OnShaft2 -> TrsmNrGear.TrsmNrGearProc.GearEvenProc.ErrCluCnt11 [order 2] : [Cntr<=0]
        TrsmNrGear.TrsmNrGearProc.GearEvenProc.ErrCluCnt11 -> TrsmNrGear.TrsmNrGearProc.GearEvenProc.Set0OnShaft2 [order 1] : [ErrCntGear<4]
        TrsmNrGear.TrsmNrGearProc.GearEvenProc.Clu1EngdClu2Disengd -> TrsmNrGear.TrsmNrGearProc.GearEvenProc.ErrCluCnt10 [order 2] : [Cntr<=0]
        TrsmNrGear.TrsmNrGearProc.GearEvenProc.ErrCluCnt10 -> TrsmNrGear.TrsmNrGearProc.GearEvenProc.Clu1EngdClu2Disengd [order 1] : [ErrCntGear<40]
        TrsmNrGear.TrsmNrGearProc.GearEvenProc.Set0OnShaft2 -> (junction 401) [order 1] : [Shaft2GearAct==0]
            | {TrsmNrGearAct=TrsmNrGearReqLocl;
            | TrsmNrPreGearAct=TrsmNrGearAct;
            | ErrCntGear=0;}
        TrsmNrGear.TrsmNrGearProc.GearEvenProc.ChkPreGearOnShaft1 -> TrsmNrGear.TrsmNrGearProc.GearEvenProc.Clu1EngdClu2Disengd [order 1] : [TrsmNrPreGearAct==TrsmNrGearReqLocl||...
            | Shaft1GearAct==TrsmNrGearReqLocl]
            | {TrsmNrPreGearAct=TrsmNrGearReqLocl;
            | ErrCntGear=0;}
        (junction 402) -> TrsmNrGear.TrsmNrGearProc.GearEvenProc.ChkPreGearOnShaft1 [order 1] : [TrsmNrGearReqLocl==1||...
            | TrsmNrGearReqLocl==3||...
            | TrsmNrGearReqLocl==5]
            | {ErrCntGear=0;}
        TrsmNrGear.TrsmNrGearProc.GearEvenProc.Clu1EngdClu2Disengd -> TrsmNrGear.TrsmNrGearProc.GearEvenProc.Set0OnShaft2 [order 1] : [Clu1Act==1&&Clu2Act==0]
            | {ErrCntGear=0;}
        (junction 401) -> (junction 404)
        (junction 402) -> (junction 403) [order 2]
        (junction 403) -> (junction 404) : {TrsmNrGearErrNr=26;}
      state GearRvsProc [group]
        state ErrCluCnt4
          en:ErrCntGear++;
        state Clu1DisengdClu2Disengd
          en:Clu1Req=0;
          Clu2Req=0;
          Cntr=10;
          du:Cntr--;
        (junction 478) -> (junction 479)
        (junction 479) -> (junction 480) : {ErrCntGear=0;}
        TrsmNrGear.TrsmNrGearProc.GearRvsProc.ErrCluCnt4 -> (junction 478) [order 2] : {TrsmNrGearErrNr=27;}
        (junction 480) -> (junction 482)
        TrsmNrGear.TrsmNrGearProc.GearRvsProc.Clu1DisengdClu2Disengd -> TrsmNrGear.TrsmNrGearProc.GearRvsProc.ErrCluCnt4 [order 2] : [Cntr<=0]
        TrsmNrGear.TrsmNrGearProc.GearRvsProc.ErrCluCnt4 -> TrsmNrGear.TrsmNrGearProc.GearRvsProc.Clu1DisengdClu2Disengd [order 1] : [ErrCntGear<40]
        (junction 481) -> TrsmNrGear.TrsmNrGearProc.GearRvsProc.Clu1DisengdClu2Disengd [order 1] : [TrsmNrGearReqLocl==0]
            | {ErrCntGear=0;}
        TrsmNrGear.TrsmNrGearProc.GearRvsProc.Clu1DisengdClu2Disengd -> (junction 1938) [order 1] : [Clu1Act==0&&Clu2Act==0]
            | {ErrCntGear=0;}
        (junction 1938) -> (junction 482) : {TrsmNrGearAct=TrsmNrGearReqLocl;
            | ErrCntGear=0;}
        (junction 481) -> (junction 483) [order 2]
        (junction 482) -> (junction 484)
        (junction 483) -> (junction 484) [order 1] : [TrsmNrGearReqLocl==7]
        (junction 483) -> (junction 1652) [order 2]
        (junction 484) -> (junction 1655)
        (junction 1652) -> (junction 1655) : {TrsmNrGearErrNr=29;}
      state end
      (junction 235) -> (junction 183)
      (default) -> TrsmNrGear.TrsmNrGearProc.Ready
      (junction 183) -> (junction 185)
      TrsmNrGear.TrsmNrGearProc.Ready -> (junction 389) [order 3] : [TrsmNrGearAct==2||...
          | TrsmNrGearAct==4||...
          | TrsmNrGearAct==6]
      TrsmNrGear.TrsmNrGearProc.Ready -> (junction 297) [order 2] : [TrsmNrGearAct==1||...
          | TrsmNrGearAct==3||...
          | TrsmNrGearAct==5]
      TrsmNrGear.TrsmNrGearProc.Ready -> (junction 221) [order 1] : [TrsmNrGearAct==0]
      TrsmNrGear.TrsmNrGearProc.Ready -> (junction 481) [order 4] : [TrsmNrGearAct==7]
      (junction 312) -> (junction 185)
      (junction 1655) -> (junction 188)
      (junction 404) -> (junction 187)
      (junction 185) -> (junction 187)
      (junction 187) -> (junction 188)
      (junction 188) -> (junction 191)
      TrsmNrGear.TrsmNrGearProc.Ready -> TrsmNrGear.TrsmNrGearProc.end [order 5] : {TrsmNrGearErrNr=1;}
      (junction 191) -> TrsmNrGear.TrsmNrGearProc.end
      TrsmNrGear.TrsmNrGearProc.end -> TrsmNrGearProc [order 1] : [TrsmNrGearErrNr>0]
          | {TrsmNrGearErr++;
          | TrsmNrGearErrNr=0;}
    (default) -> TrsmNrGearStdySt
    TrsmNrGearStdySt -> TrsmNrGearProc : [TrsmNrGearReq!=TrsmNrGearAct&&...
        | PreGearShiftFlg==0]
    TrsmNrGearProc -> TrsmNrGearProc : [TrsmNrGearReq!=TrsmNrGearReqLocl&&...
        | TrsmNrGearReq==0]
        | {TrsmNrGearAct=TrsmNrGearReqLocl;}
    TrsmNrGear.TrsmNrGearProc.end -> TrsmNrGearStdySt [order 2] : [TrsmNrGearAct==TrsmNrGearReqLocl]
        | {GearShiftFlg=0;}
  data: Shaft1GearReq output uint8 [0..8] =0; Shaft2GearReq output uint8 =0; Clu1Req output uint8 =0; Clu2Req output uint8 =0; TrsmNrGearAct output uint8 [0..8] =0; TrsmNrPreGearAct output uint8 =0; TrsmNrPreGearReqLocl local uint8 [0..8]; TrsmNrGearReqLocl local uint8 [0..8]; ErrCntShaft local uint8; GearShiftFlg local uint8; PreGearShiftFlg local uint8; Cntr local uint8; ErrCntGear local uint8; TrsmNrPreGearReq input uint8; TrsmNrGearReq input uint8; Shaft1GearAct input uint8 [0..8]; Shaft2GearAct input uint8 [0..8]; Clu1Act input uint8; Clu2Act input uint8; TrsmNrGearErrNr local uint8; TrsmNrPreGearErrNr local uint8; TrsmNrGearErr output uint8 =0; TrsmNrPreGearErr output uint8 =0; BrkSig input uint8
